simulink model "formation_control_2N"  (R2021a)
settings: Solver=VariableStepAuto  StartTime=0.0  StopTime=T  RelTol=1e-3
undefined symbols (not defined in the file or in its folder): params
settings Model: Creator=gaeta  LastModifiedBy=giuse
settings SolverCC: AlgebraicLoopSolver=TrustRegion
settings DataIOCC: InitialState=initialCondition  LoadInitialState=on
settings DebuggingCC: SFMachineParentedDataDiag=warning

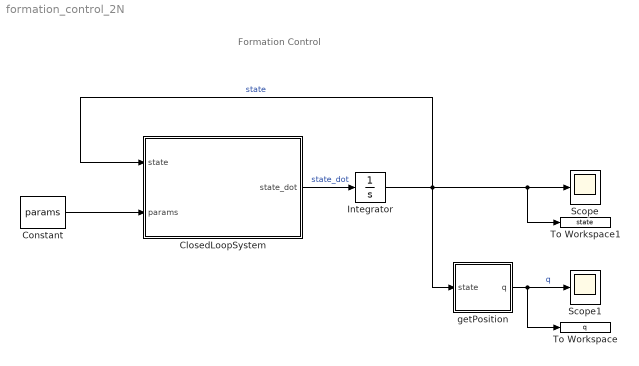
== system formation_control_2N ==
  note: Formation Control
  ClosedLoopSystem : MATLAB Function  TreatAsAtomicUnit=on
  Constant : Constant  Value=params  OutDataTypeStr=Bus: params_bus
  Integrator : Integrator
  Scope : Scope
  Scope1 : Scope
  To Workspace : ToWorkspace  VariableName=q  SaveFormat=Timeseries  SampleTime=-1
  To Workspace1 : ToWorkspace  VariableName=state  SaveFormat=Timeseries  SampleTime=-1
  getPosition : Subsystem
  wires:
  Constant/1 -> ClosedLoopSystem/2(params)
  Integrator/1 -> getPosition/1(state), To Workspace1/1, Scope/1, ClosedLoopSystem/1(state)  "state"
  ClosedLoopSystem/1(state_dot) -> Integrator/1  "state_dot"
  getPosition/1(q) -> To Workspace/1, Scope1/1  "q"

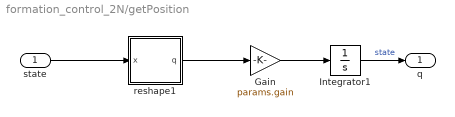
== system formation_control_2N/getPosition ==
  state : Inport
  Gain : Gain  Gain=params.gain
  Integrator1 : Integrator
  reshape1 : MATLAB Function  TreatAsAtomicUnit=on
  q : Outport
  wires:
  state/1 -> reshape1/1(x)
  reshape1/1(q) -> Gain/1
  Gain/1 -> Integrator1/1
  Integrator1/1 -> q/1  "state"

== matlab function formation_control_2N/getPosition/reshape1 ==
  data: q output size=params.N*3; x input
function q = reshape(x)
    q = x(1:6);
end




%

== matlab function formation_control_2N/ClosedLoopSystem ==
  data: state input size=3*(params.N+params.E); state_dot output size=3*(params.N+params.E); params input
function state_dot = ClosedLoopSystem(state,params)

    n = 3;                      % task space
    N = params.N;               % number of robots
    
    p = state(1:n*N);           % robots momenta
    m = params.m;               % robots masses
    M = zeros(n*N, n*N);      	% inertia matrix
    d = params.d;               % frict. coeff
    D = zeros(n*N, n*N);        % system dissipation matrix
    for i = 1:N
        M(n*i-n+1:n*i, n*i-n+1:n*i) = eye(n).*m(i);
        D(n*i-n+1:n*i, n*i-n+1:n*i) = eye(n).*d(i);
    end
    
	E = params.E;           % number of edges
    B = params.B            % incidence matrix
    Bcl = kron(B,eye(n));	% closed-loop incidence matrix    

    z = state(n*N+1:n*(N+E));      % edges lengths
    z_des = params.z_des;   % desired edges lengths
    dc = params.dc;         % robots dissipations
    Dc = zeros(n*E, n*E);	% controller dissipation matrix
    kc = params.kc;         % constant springs
    Kc = zeros(n*E, n*E);	% constant spring matrix
    for j = 1:E
        Dc(n*j-n+1:n*j, n*j-n+1:n*j) = eye(n).*dc(j);
        Kc(n*j-n+1:n*j, n*j-n+1:n*j) = eye(n).*kc(j);
    end

    p_dot = [-(D + Bcl*Dc*Bcl.'), -Bcl] * [M^-1*p; Kc*(z-z_des)];
    z_dot = Bcl.' * M^-1*p;

    state_dot = [p_dot; z_dot]
end




%
